simulink model "simulink_1"  (R2016b)
settings: Solver=VariableStepAuto  StartTime=0.0  StopTime=10.0  RelTol=1e-3
settings Model: Creator=XPS  LastModifiedBy=XPS

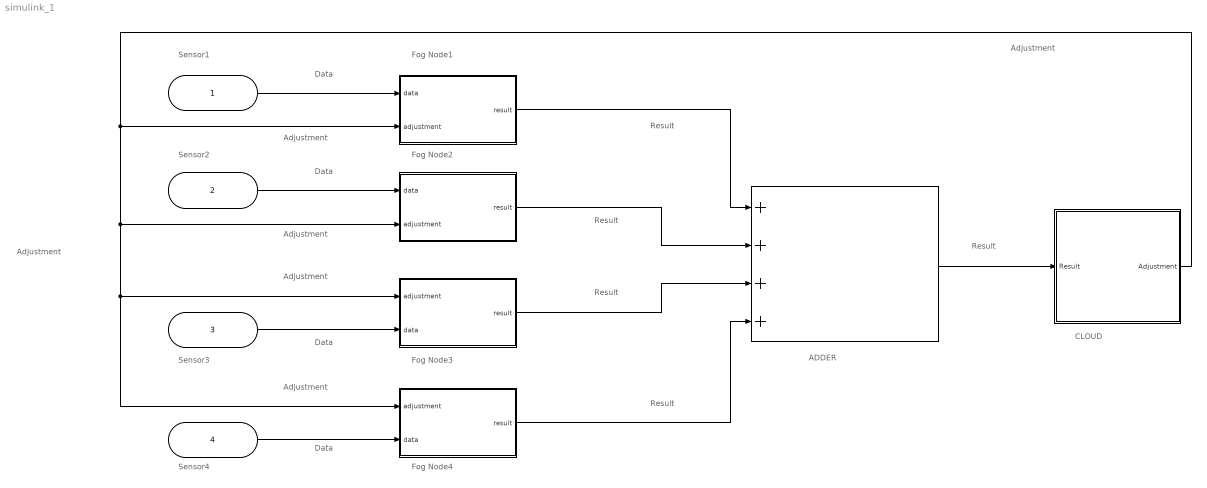
== system simulink_1 ==
  note: Result
  note: Adjustment
  note: ADDER
  note: CLOUD
  note: Fog Node1
  note: Fog Node2
  note: Fog Node3
  note: Fog Node4
  note: Sensor1
  note: Sensor2
  note: Sensor3
  note: Sensor4
  note: Adjustment
  note: Adjustment
  note: Adjustment
  note: Adjustment
  note: Adjustment
  note: Data
  note: Data
  note: Data
  note: Data
  note: Result
  note: Result
  note: Result
  note: Result
  "                                          " : Inport
  " " : Inport  Port=2
  "                                              " : Inport  Port=3
  " " : Inport  Port=4
  " " : Sum  Inputs=4
  " " : Subsystem
  " " : MATLAB Function  TreatAsAtomicUnit=on
  "      " : MATLAB Function  TreatAsAtomicUnit=on
  "         " : MATLAB Function  TreatAsAtomicUnit=on
  "             " : MATLAB Function  TreatAsAtomicUnit=on
  wires:
  "                                          "/1 -> " "/1(data)
  " "/1 -> "      "/1(data)
  " "/1 -> "             "/2(data)
  " "/1(result) -> " "/1
  "      "/1(result) -> " "/2
  "         "/1(result) -> " "/3
  "             "/1(result) -> " "/4
  " "/1 -> " "/1(Result)
  " "/1(Adjustment) -> " "/2(adjustment), "      "/2(adjustment), "         "/1(adjustment), "             "/1(adjustment)
  "                                              "/1 -> "         "/2(data)

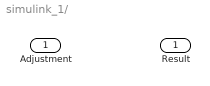
== system simulink_1/  ==
  Result : Inport
  Adjustment : Outport

== matlab function simulink_1/       ==
  data: data input; result output; adjustment input
function result = fcn(data,adjustment)

result= data;

== matlab function simulink_1/  ==
  data: data input; result output; adjustment input
function result = fcn(data,adjustment)

result= data;

== matlab function simulink_1/          ==
  data: adjustment input; data input; result output
function result = fcn(adjustment,data)

result= data;

== matlab function simulink_1/              ==
  data: adjustment input; data input; result output
function result = fcn(adjustment,data)

result= data;
